simulink model "P2_B0"  (R2018a)
settings: Solver=VariableStepAuto  StartTime=0.0  StopTime=15.0  RelTol=1e-3
settings Model: Creator=Erfan Panahi  LastModifiedBy=Erfan Panahi

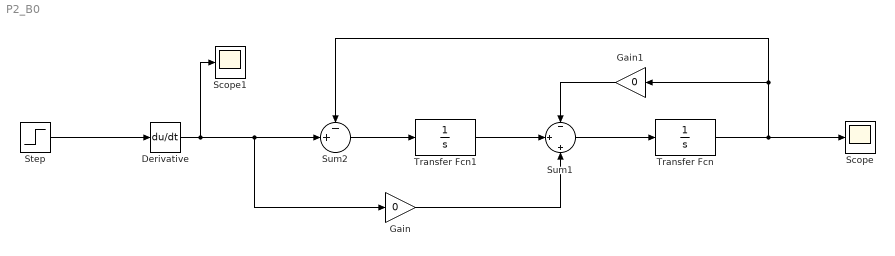
== system P2_B0 ==
  Derivative : Derivative
  Gain : Gain  Gain=0
  Gain1 : Gain  Gain=0
  Scope : Scope
  Scope1 : Scope
  Step : Step  Time=0.001  SampleTime=0
  Sum1 : Sum  Inputs=-|+|+
  Sum2 : Sum  Inputs=-+|
  Transfer Fcn : TransferFcn  Denominator=[1 0]
  Transfer Fcn1 : TransferFcn  Denominator=[1 0]
  wires:
  Transfer Fcn/1 -> Gain1/1, Sum2/1, Scope/1
  Sum2/1 -> Transfer Fcn1/1
  Step/1 -> Derivative/1
  Transfer Fcn1/1 -> Sum1/2
  Sum1/1 -> Transfer Fcn/1
  Derivative/1 -> Gain/1, Sum2/2, Scope1/1
  Gain1/1 -> Sum1/1
  Gain/1 -> Sum1/3
